simulink model "Logan"  (R2024b)
settings: Solver=ode4  StartTime=0  StopTime=inf  FixedStep=0.01  RelTol=1e-3
values from neighbouring files (symbols this model uses):
  AltPoint = 100000    [Logan_init.m]
  area_secao = 79.402*1.5    (= 119.103)    [Logan_init.m]
  b = 9    [Logan_init.m]
  c = 15.252    [Logan_init.m]
  cp = 1003    [Logan_init.m]
  E = 110e9    (= 110000000000)    [Logan_init.m]
  eta_comb = 0.95    [Logan_init.m]
  Fuel_Freeze = 0    [Logan_init.m]
  g = 9.80665    [Logan_init.m]
  gamma = 1.4    [Logan_init.m]
  GammaRef_deg = 0    [Logan_init.m]
  h1 = 0.5746    [Logan_init.m]
  h2 = 0.7752    [Logan_init.m]
  h3 = 0.1502    [Logan_init.m]
  hc = h1 + h2 + h3    (= 1.5)    [Logan_init.m]
  he = 2.6    [Logan_init.m]
  Inertia = [Ixx 0 -Ixz; 0 Iyy 0; -Ixz 0 Izz]    [Logan_init.m]
  L = 22.5    [Logan_init.m]
  L_inlet = 5.5    [Logan_init.m]
  La = 5    [Logan_init.m]
  LHV = 120 * 10^6    (= 120000000)    [Logan_init.m]
  Ln0 = 4.8    [Logan_init.m]
  MachPoint = 10    [Logan_init.m]
  Manual_Control = 0    [Logan_init.m]
  MW_air = 28.85    [Logan_init.m]
  MW_H2 = 2.00    (= 2)    [Logan_init.m]
  PA_EngineMode = 0    [Logan_init.m]
  PA_LatMode = 2    [Logan_init.m]
  PA_LongMode = 2    [Logan_init.m]
  PA_TECSEngineInput = 0    [Logan_init.m]
  PhiPoint = 0    [Logan_init.m]
  R = 287    [Logan_init.m]
  RefMass_kg = 31000    [Logan_init.m]
  S = 91.5    [Logan_init.m]
  tau1 = 3.1    [Logan_init.m]
  tau2 = 18.23    [Logan_init.m]
  TECS_ON = 0    [Logan_init.m]
  theta1 = 4    [Logan_init.m]
  theta2 = 6    [Logan_init.m]
  theta_n = 4    [Logan_init.m]
  ThetaPoint = 0    [Logan_init.m]
  Trimming = 0    [Logan_init.m]    (also in Logan_trim.m)
  w = 3.000    (= 3)    [Logan_init.m]
  Waypoint_idx = 1    [Logan_init.m]
  Waypoints = [ ... (first row only)    [Logan_init.m]
  x_a = 3.7    [Logan_init.m]
  x_inlet = 6    [Logan_init.m]
  x_n0 = 3    [Logan_init.m]
  xf_m = 0    [Logan_init.m]
  y_cg = 0    [Logan_init.m]
  z_a = 0.4    [Logan_init.m]
  z_cg = -0.996    [Logan_init.m]
  z_inlet = 0.7    [Logan_init.m]
  zf_m = 0    [Logan_init.m]
undefined symbols (not defined in the file or in its folder): Earth, Receive, Send, WGS84
libraries: simulink x4, spsFirstOrderFilterLib x4, aerolibactuator x3, aerolibfltsims x2, aerolibatmos2 x1, aerolibtransform2 x1, aerolibanimutils x1, dspswit3 x1, spsEdgeDetectorLib x1
(part 1 of 5)
settings Model: PacingRate=1000  Creator=bruno  LastModifiedBy=Ermer
settings SolverCC: NumberNewtonIterations=10  AlgebraicLoopSolver=TrustRegion
settings DataIOCC: ExternalInput=getinputstruct(opreport)  InitialState=getstatestruct(opreport)  LoadExternalInput=on  LoadInitialState=on  SaveFormat=StructureWithTime  ReturnWorkspaceOutputs=off
settings OptimizationCC: BlockReduction=off  DefaultParameterBehavior=Inlined  OptimizeBlockIOStorage=off  BufferReuse=off  EnhancedBackFolding=on  PassReuseOutputArgsAs=Individual arguments  ZeroExternalMemoryAtStartup=off  ZeroInternalMemoryAtStartup=off  OptimizeBlockOrder=speed  DifferentSizesBufferReuse=on  EfficientTunableParamExpr=on
settings DebuggingCC: AlgebraicLoopMsg=none  ParameterTunabilityLossMsg=error  SFUnexpectedBacktrackingDiag=warning  SFNoUnconditionalDefaultTransitionDiag=warning  ArithmeticOperatorsInVariantConditions=warning
settings ModelReferenceCC: EnableRefExpFcnMdlSchedulingChecks=on
settings SFSimCC: SimUseLocalCustomCode=off  MATLABDynamicMemAlloc=off  CustomCodeUndefinedFunction=UseInterfaceOnly
settings RTWCC: Description=Embedded Coder  SystemTargetFile=ert.tlc  TemplateMakefile=ert_default_tmf  RTWUseLocalCustomCode=off  GPUComputeCapability=3.5
settings CodeAppCC: ForceParamTrailComments=on  IgnoreCustomStorageClasses=off  OperatorAnnotations=on  SimulinkDataObjDesc=on  SFDataObjDesc=on  InsertBlockDesc=on
settings ERTTargetCC: GenerateSampleERTMain=on  SupportContinuousTime=on  ERTCustomFileTemplate=example_file_process.tlc  DynamicArrayContainerType=coder::array
settings ConfigComp: CovMetricSettings=dw  CovSaveCumulativeToWorkspaceVar=on  CovSaveSingleToWorkspaceVar=on  CovExternalEMLEnable=off
settings ExplorerConfigSet: SimMechanicsOpenEditorOnUpdate=off

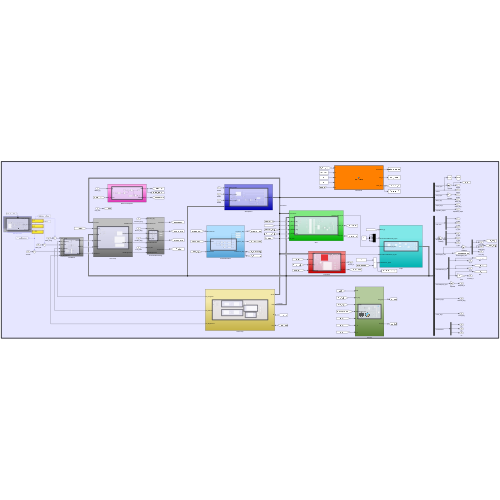
[thumbnail: Simulink's stored preview of the top-level diagram]
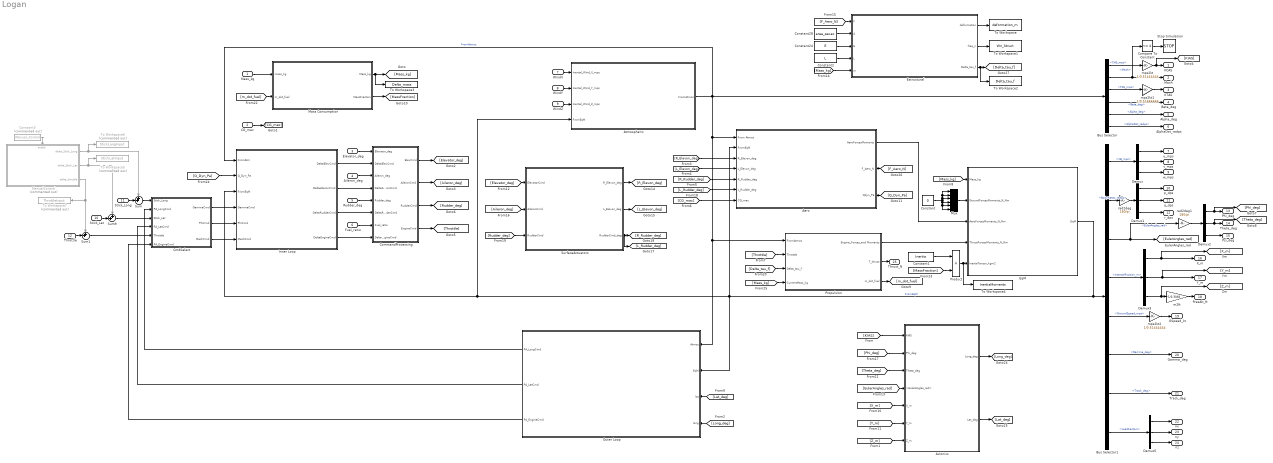
== system Logan ==
  Mass_kg : Inport  OutDataTypeStr=double
  CG_mac : Inport  Port=2  OutDataTypeStr=double
  Elevator_deg : Inport  Port=3  OutDataTypeStr=double
  Aileron_deg : Inport  Port=4  OutDataTypeStr=double
  Rudder_deg : Inport  Port=5  OutDataTypeStr=double
  Fuel_ratio : Inport  Port=6  OutDataTypeStr=double
  WindX : Inport  Port=7  OutDataTypeStr=double
  WindY : Inport  Port=8  OutDataTypeStr=double
  WindZ : Inport  Port=9  OutDataTypeStr=double
  Stick_Lat : Inport  Port=10
  Stick_Long : Inport  Port=11
  Throttle : Inport  Port=12  OutDataTypeStr=double
  Aero : Subsystem
  Atmospheric : Subsystem
  Avionics : Subsystem
  Bus Selector : BusSelector  OutputSignals=CAS_mps,Mach,TAS_mps,Beta_deg,Alpha_deg,AlphaDot_radps
  Bus Selector1 : BusSelector  OutputSignals=VB_mps,BodyRates_radps,EulerAngles_rad,IntertialPosition_m,GroundSpeed_mps,Gamma_deg,Track_deg,LoadFactors
  CmdSelect : Subsystem
  CommandProcessing : Subsystem
  Compare To Constant : simulink/Logic and Bit Operations/Compare To Constant  relop=<=  const=4  OutDataTypeStr=boolean
  Constant : Constant  Value=0  OutDataTypeStr=double
  Constant1 : Constant  Value=Inertia  OutDataTypeStr=double
  Constant2 : Constant  Value=L
  Constant24 : Constant  Value=E
  Constant28 : Constant  Value=area_secao
  Constant3 : Constant  Commented=on  Value=Manual_Control
  Demux{,1..3,5} (5 alike) : Demux  Outputs=3
  EqM : Subsystem
  Estructural : MATLAB Function  TreatAsAtomicUnit=on
  Inner Loop : Subsystem
  ManualControl : Subsystem  Commented=on
  Mass Consumption : Subsystem
  Mux : Mux  Inputs=6
  Outer Loop : Subsystem
  Product : Product
  Propulsion : Subsystem
  Stop Simulation : Stop
  Sum : Sum  Inputs=++|
  Sum1 : Sum  Inputs=++|
  Sum9 : Sum  Inputs=++|
  SurfaceActuators : Subsystem
  To Workspace : ToWorkspace  VariableName=deformation_m  SampleTime=-1
      settings: Save2DSignal=2-D array (concatenate along first dimension)
  To Workspace1 : ToWorkspace  VariableName=Wn_Struct  SampleTime=-1
      settings: Save2DSignal=2-D array (concatenate along first dimension)
  To Workspace2 : ToWorkspace  VariableName=Delta_tau_f  SampleTime=-1
  To Workspace3 : ToWorkspace  VariableName=Delta_mass  SampleTime=-1
      settings: Save2DSignal=2-D array (concatenate along first dimension)
  To Workspace4 : ToWorkspace  VariableName=InertiaMoments  SampleTime=-1
  To Workspace5 : ToWorkspace  Commented=on  VariableName=StickLatInput  SampleTime=-1
      settings: Save2DSignal=2-D array (concatenate along first dimension)
  To Workspace6 : ToWorkspace  Commented=on  VariableName=StickLongInput  SampleTime=-1
      settings: Save2DSignal=2-D array (concatenate along first dimension)
  To Workspace7 : ToWorkspace  Commented=on  VariableName=ThrottleInput  SampleTime=-1
      settings: Save2DSignal=2-D array (concatenate along first dimension)
  m2ft : Gain  Gain=-1/0.3048
  mps2kt : Gain  Gain=1/0.51444444
  mps2kt1 : Gain  Gain=1/0.51444444
  mps2kt2 : Gain  Gain=1/0.51444444
  rad2deg : Gain  Gain=180/pi
  rad2deg1 : Gain  Gain=180/pi
  KCAS : Outport
  Mach : Outport  Port=2
  KTAS : Outport  Port=3
  Beta_deg : Outport  Port=4
  Alpha_deg : Outport  Port=5
  AlphaDot_radps : Outport  Port=6
  u_mps : Outport  Port=7
  v_mps : Outport  Port=8
  w_mps : Outport  Port=9
  p_dps : Outport  Port=10
  q_dps : Outport  Port=11
  r_dps : Outport  Port=12
  Phi_deg : Outport  Port=13
  Theta_deg : Outport  Port=14
  Psi_deg : Outport  Port=15
  X_m : Outport  Port=16
  Y_m : Outport  Port=17
  PresAlt_ft : Outport  Port=18
  GSpeed_kt : Outport  Port=19
  Gamma_deg : Outport  Port=20
  Track_deg : Outport  Port=21
  nx : Outport  Port=22
  ny : Outport  Port=23
  nz : Outport  Port=24
  Thrust_N : Outport  Port=25
  wires:
  Atmospheric/1(FromAtmos) -> Outer Loop/1(Atmos), Propulsion/1(FromAtmos), Aero/1(From Atmos), Inner Loop/1(FromAtm), Bus Selector/1  "FromAtmos"
  Aero/1(AeroForcesMoments) -> EqM/3(AeroForcesMoments_N_Nm)
  Propulsion/1(Engine_Forces_and Moments) -> EqM/4(ThrustForcesMoments_N_Nm)
  EqM/1(EqM) -> Outer Loop/2(EqM), Inner Loop/3(FromEqM), Atmospheric/4(FromEqM), Aero/2(FromEqM), Bus Selector1/1  "FromEqM"
  Constant/1 -> Mux/4, Mux/5, Mux/6, Mux/2, Mux/1, Mux/3
  Mux/1 -> EqM/2(GroundForcesMoments_N_Nm)
  CG_mac/1 -> [CG_mac]
  WindX/1 -> Atmospheric/1(Inertial_Wind_X_mps)
  WindY/1 -> Atmospheric/2(Inertial_Wind_Y_mps)
  WindZ/1 -> Atmospheric/3(Inertial_Wind_Z_mps)
  [R_Elevon_deg] -> Aero/3(R_Elevon_deg)
  [L_Elevon_deg] -> Aero/4(L_Elevon_deg)
  [R_Rudder_deg] -> Aero/5(R_Rudder_deg)
  [CG_mac] -> Aero/7(CG_mac)
  [Mass_kg] -> EqM/1(Mass_kg)
  Propulsion/2(T_thrust) -> Thrust_N/1
  Bus Selector/1 -> mps2kt/1  "<CAS_mps>"
  Bus Selector/2 -> Compare To Constant/1, Mach/1  "<Mach>"
  Bus Selector/3 -> mps2kt1/1  "<TAS_mps>"
  mps2kt1/1 -> KTAS/1
  Bus Selector/4 -> Beta_deg/1  "<Beta_deg>"
  Bus Selector/5 -> Alpha_deg/1  "<Alpha_deg>"
  Bus Selector/6 -> AlphaDot_radps/1  "<AlphaDot_radps>"
  Bus Selector1/1 -> Demux/1  "<VB_mps>"
  Demux/1 -> u_mps/1
  Demux/2 -> v_mps/1
  Demux/3 -> w_mps/1
  Bus Selector1/2 -> rad2deg/1  "<BodyRates_radps>"
  Demux1/1 -> p_dps/1
  Demux1/3 -> r_dps/1
  Bus Selector1/3 -> rad2deg1/1, [EulerAngles_rad]  "<EulerAngles_rad>"
  Demux2/2 -> Theta_deg/1, [Theta_deg]
  Demux2/3 -> Psi_deg/1
  rad2deg/1 -> Demux1/1
  rad2deg1/1 -> Demux2/1
  Bus Selector1/4 -> Demux3/1  "<IntertialPosition_m>"
  Demux3/1 -> X_m/1, [X_m]
  Demux3/2 -> Y_m/1, [Y_m]
  Demux3/3 -> [Z_m], m2ft/1
  m2ft/1 -> PresAlt_ft/1
  Bus Selector1/5 -> mps2kt2/1  "<GroundSpeed_mps>"
  mps2kt2/1 -> GSpeed_kt/1
  Bus Selector1/6 -> Gamma_deg/1  "<Gamma_deg>"
  Bus Selector1/7 -> Track_deg/1  "<Track_deg>"
  Bus Selector1/8 -> Demux5/1  "<LoadFactors>"
  Demux5/1 -> nx/1
  Demux5/2 -> ny/1
  Demux5/3 -> nz/1
  [Throttle] -> Propulsion/2(Throttle)
  mps2kt/1 -> KCAS/1, [KIAS]
  Demux1/2 -> q_dps/1
  [L_Rudder_deg] -> Aero/6(L_Rudder_deg)
  Estructural/1(deformation) -> To Workspace/1
  Estructural/2(freq_n) -> To Workspace1/1
  Avionics/1(Long_deg) -> [Long_deg]
  Avionics/2(Lat_deg) -> [Lat_deg]
  [Mass_kg] -> Estructural/5(m)
  Constant2/1 -> Estructural/4(L)
  Constant24/1 -> Estructural/3(E)
  Constant28/1 -> Estructural/2(A)
  Aero/2(F_Aero_N) -> [F_Aero_N]
  [F_Aero_N] -> Estructural/1(F)
  Estructural/3(Delta_tau_f) -> To Workspace2/1, [Delta_tau_f]
  [Delta_tau_f] -> Propulsion/3(Delta_tau_f)
  SurfaceActuators/1(R_Elevon_deg) -> [R_Elevon_deg]
  SurfaceActuators/2(L_Elevon_deg) -> [L_Elevon_deg]
  [Aileron_deg] -> SurfaceActuators/2(AileronCmd)
  [Elevator_deg] -> SurfaceActuators/1(ElevatorCmd)
  [Rudder_deg] -> SurfaceActuators/3(RudderCmd)
  SurfaceActuators/3(RudderCmd_deg) -> [R_Rudder_deg], [L_Rudder_deg]
  Elevator_deg/1 -> CommandProcessing/1(Elevator_deg)
  Inner Loop/1(DeltaElevCmd) -> CommandProcessing/2(DeltaElevCmd)
  CmdSelect/1(GammaCmd) -> Inner Loop/4(GammaCmd)
  Constant3/1 -> ManualControl/Enable
  Stick_Long/1 -> Sum/2
  Sum/1 -> CmdSelect/1(Stick_Long)
  ManualControl/1(delta_Stick_Long) -> To Workspace6/1, Sum/1
  Inner Loop/2(DeltaAileronCmd) -> CommandProcessing/4(DeltaAileronCmd)
  Inner Loop/3(DeltaRudderCmd) -> CommandProcessing/6(DeltaRudderCmd)
  CommandProcessing/3(RudderCmd) -> [Rudder_deg]
  Rudder_deg/1 -> CommandProcessing/5(Rudder_deg)
  CommandProcessing/2(AileronCmd) -> [Aileron_deg]
  Aileron_deg/1 -> CommandProcessing/3(Aileron_deg)
  Sum9/1 -> CmdSelect/3(Stick_Lat)
  Stick_Lat/1 -> Sum9/2
  ManualControl/2(delta_Stick_Lat) -> To Workspace5/1, Sum9/1
  CmdSelect/2(PhiCmd) -> Inner Loop/5(PhiCmd)
  CmdSelect/3(MachCmd) -> Inner Loop/6(MachCmd)
  ManualControl/3(delta_throttle) -> Sum1/1, To Workspace7/1
  Sum1/1 -> CmdSelect/5(Throttle)
  Outer Loop/1(PA_LongCmd) -> CmdSelect/2(PA_LongCmd)
  Outer Loop/2(PA_LatCmd) -> CmdSelect/4(PA_LatCmd)
  [Lat_deg] -> Outer Loop/3(lat)
  [Long_deg] -> Outer Loop/4(long)
  [Z_m] -> Avionics/7(Z_m)
  [KIAS] -> Avionics/1(KIAS)
  [X_m] -> Avionics/5(X_m)
  [Y_m] -> Avionics/6(Y_m)
  [EulerAngles_rad] -> Avionics/4(<EulerAngles_rad>)
  [Phi_deg] -> Avionics/2(Phi_deg)
  [Theta_deg] -> Avionics/3(Theta_deg)
  Demux2/1 -> Phi_deg/1, [Phi_deg]
  Outer Loop/3(PA_EngineCmd) -> CmdSelect/6(PA_EngineCmd)
  Throttle/1 -> Sum1/2
  CommandProcessing/4(EngineCmd) -> [Throttle]
  Inner Loop/4(DeltaEngineCmd) -> CommandProcessing/8(DeltaEngineCmd)
  Fuel_ratio/1 -> CommandProcessing/7(Fuel_ratio)
  CommandProcessing/1(ElevCmd) -> [Elevator_deg]
  Propulsion/3(m_dot_fuel) -> [m_dot_fuel]
  Mass_kg/1 -> Mass Consumption/1(mass_kg)
  Mass Consumption/1(Mass_kg) -> To Workspace3/1, [Mass_kg]
  [m_dot_fuel] -> Mass Consumption/2(m_dot_fuel)
  Mass Consumption/2(MassFraction) -> [MassFraction]
  Product/1 -> To Workspace4/1, EqM/5(InertiaTensor_kgm2)
  Constant1/1 -> Product/1
  [MassFraction] -> Product/2
  [Mass_kg] -> Propulsion/4(CurrentMass_kg)
  Compare To Constant/1 -> Stop Simulation/1
  Aero/3(Qdyn_Pa) -> [Q_Dyn_Pa]
  [Q_Dyn_Pa] -> Inner Loop/2(Q_Dyn_Pa)

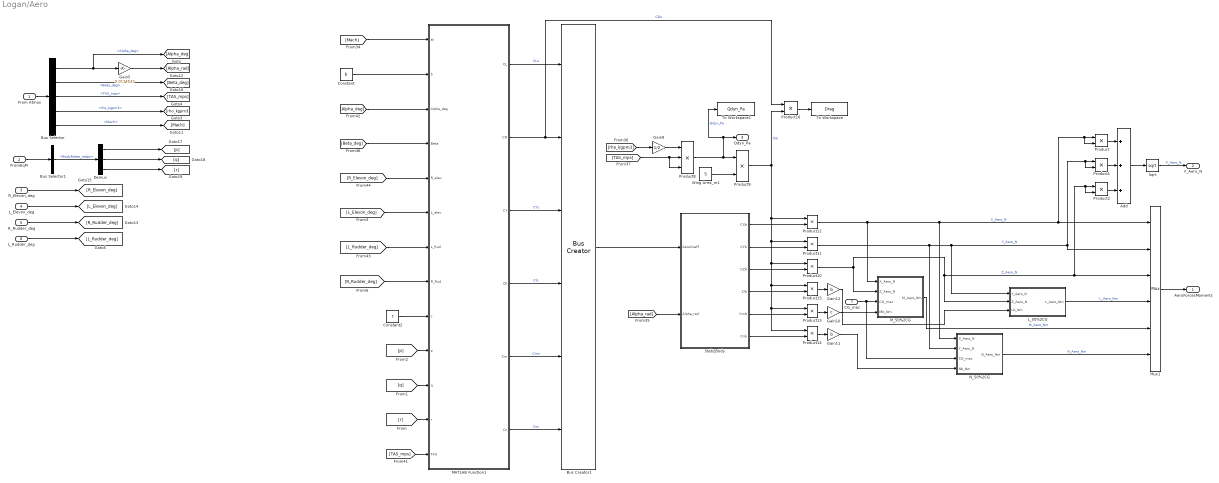
== system Logan/Aero ==
  From Atmos : Inport
  FromEqM : Inport  Port=2
  R_Elevon_deg : Inport  Port=3
  L_Elevon_deg : Inport  Port=4
  R_Rudder_deg : Inport  Port=5
  L_Rudder_deg : Inport  Port=6
  CG_mac : Inport  Port=7
  Add : Sum  Inputs=+++
  Bus Creator1 : BusCreator  Inputs=6
  Bus Selector : BusSelector  OutputSignals=Alpha_deg,Beta_deg,TAS_mps,rho_kgpm3,Mach
  Bus Selector1 : BusSelector  OutputSignals=BodyRates_radps
  Constant : Constant  Value=b
  Constant2 : Constant  Value=c
  Demux : Demux  Outputs=3
  Gain10 : Gain  Gain=c
  Gain11 : Gain  Gain=b
  Gain12 : Gain  Gain=b
  Gain5 : Gain  Gain=0.0174533
  Gain9 : Gain  Gain=1/2
  L_50%2CG : Subsystem
  MATLAB Function1 : MATLAB Function  TreatAsAtomicUnit=on
  M_50%2CG : Subsystem
  Mux1 : Mux  Inputs=6
  N_50%2CG : Subsystem
  Product{,1..2,9..16} (11 alike) : Product
  Product8 : Product  Inputs=3
  Sqrt : Sqrt
  Stab2Body : Subsystem
  To Workspace : ToWorkspace  VariableName=Drag  SampleTime=-1
      settings: Save2DSignal=2-D array (concatenate along first dimension)
  To Workspace1 : ToWorkspace  VariableName=Qdyn_Pa  SampleTime=-1
      settings: Save2DSignal=2-D array (concatenate along first dimension)
  Wing Area_m1 : Constant  Value=S
  AeroForcesMoments : Outport
  F_Aero_N : Outport  Port=2
  Qdyn_Pa : Outport  Port=3
  wires:
  Bus Selector/4 -> [rho_kgpm3]  "<rho_kgpm3>"
  Bus Selector/3 -> [TAS_mps]  "<TAS_mps>"
  R_Rudder_deg/1 -> [R_Rudder_deg]
  Bus Selector/2 -> [Beta_deg]  "<Beta_deg>"
  L_Elevon_deg/1 -> [L_Elevon_deg]
  From Atmos/1 -> Bus Selector/1
  Bus Selector/1 -> [Alpha_deg], Gain5/1  "<Alpha_deg>"
  FromEqM/1 -> Bus Selector1/1
  Bus Selector1/1 -> Demux/1  "<BodyRates_radps>"
  Bus Selector/5 -> [Mach]  "<Mach>"
  Gain5/1 -> [Alpha_rad]
  Product15/1 -> Gain12/1
  Wing Area_m1/1 -> Product9/2
  Product10/1 -> M_50%2CG/2(Z_Aero_N), L_50%2CG/2(Z_Aero_N), Product2/2, Product2/1, Mux1/3  "Z_Aero_N"
  Product9/1 -> Product16/2, Product10/1, Product13/1, Product14/1, Product15/1, Product11/1, Product12/1  "QS"
  CG_mac/1 -> M_50%2CG/3(CG_mac), N_50%2CG/3(CG_mac)
  Product11/1 -> N_50%2CG/2(Y_Aero_N), Product1/2, Product1/1, Mux1/2, L_50%2CG/1(Y_Aero_N)  "Y_Aero_N"
  L_50%2CG/1(L_Aero_Nm) -> Mux1/4  "L_Aero_Nm"
  Product8/1 -> To Workspace1/1, Qdyn_Pa/1, Product9/1  "Qdyn_Pa"
  [TAS_mps] -> Product8/2, Product8/3
  Gain9/1 -> Product8/1
  Gain11/1 -> N_50%2CG/4(Nb_Nm)
  Product14/1 -> Gain11/1
  M_50%2CG/1(M_Aero_Nm) -> Mux1/5  "M_Aero_Nm"
  [rho_kgpm3] -> Gain9/1
  Product12/1 -> M_50%2CG/1(X_Aero_N), N_50%2CG/1(X_Aero_N), Product/2, Product/1, Mux1/1  "X_Aero_N"
  Gain10/1 -> M_50%2CG/4(Mb_Nm)
  Product13/1 -> Gain10/1
  Gain12/1 -> L_50%2CG/3(Lb_Nm)
  N_50%2CG/1(N_Aero_Nm) -> Mux1/6  "N_Aero_Nm"
  [TAS_mps] -> MATLAB Function1/13(TAS)
  [Mach] -> MATLAB Function1/1(M)
  Constant/1 -> MATLAB Function1/2(b)
  Constant2/1 -> MATLAB Function1/9(c)
  MATLAB Function1/2(CD) -> Product16/1, Bus Creator1/2  "CDs"
  MATLAB Function1/3(CY) -> Bus Creator1/3  "CYs"
  MATLAB Function1/4(Cll) -> Bus Creator1/4  "Cls"
  MATLAB Function1/5(Cm) -> Bus Creator1/5  "Cms"
  MATLAB Function1/6(Cn) -> Bus Creator1/6  "Cns"
  MATLAB Function1/1(CL) -> Bus Creator1/1  "CLs"
  Mux1/1 -> AeroForcesMoments/1
  R_Elevon_deg/1 -> [R_Elevon_deg]
  Product16/1 -> To Workspace/1
  [Alpha_rad] -> Stab2Body/2(Alpha_rad)
  Demux/1 -> [p]
  Demux/2 -> [q]
  Demux/3 -> [r]
  L_Rudder_deg/1 -> [L_Rudder_deg]
  Stab2Body/6(Cnb) -> Product14/2
  Stab2Body/5(Cmb) -> Product13/2
  Stab2Body/4(Clb) -> Product15/2
  Stab2Body/3(CZb) -> Product10/2
  Stab2Body/2(CYb) -> Product11/2
  Stab2Body/1(CXb) -> Product12/2
  Bus Creator1/1 -> Stab2Body/1(AeroCoeff)
  [r] -> MATLAB Function1/12(r)
  [Beta_deg] -> MATLAB Function1/4(Beta)
  [q] -> MATLAB Function1/11(q)
  [p] -> MATLAB Function1/10(p)
  [Alpha_deg] -> MATLAB Function1/3(Alpha_deg)
  [R_Elevon_deg] -> MATLAB Function1/5(R_elev)
  [L_Elevon_deg] -> MATLAB Function1/6(L_elev)
  [L_Rudder_deg] -> MATLAB Function1/7(L_Rud)
  [R_Rudder_deg] -> MATLAB Function1/8(R_Rud)
  Add/1 -> Sqrt/1
  Product/1 -> Add/1
  Product1/1 -> Add/2
  Product2/1 -> Add/3
  Sqrt/1 -> F_Aero_N/1  "F_Aero_N"

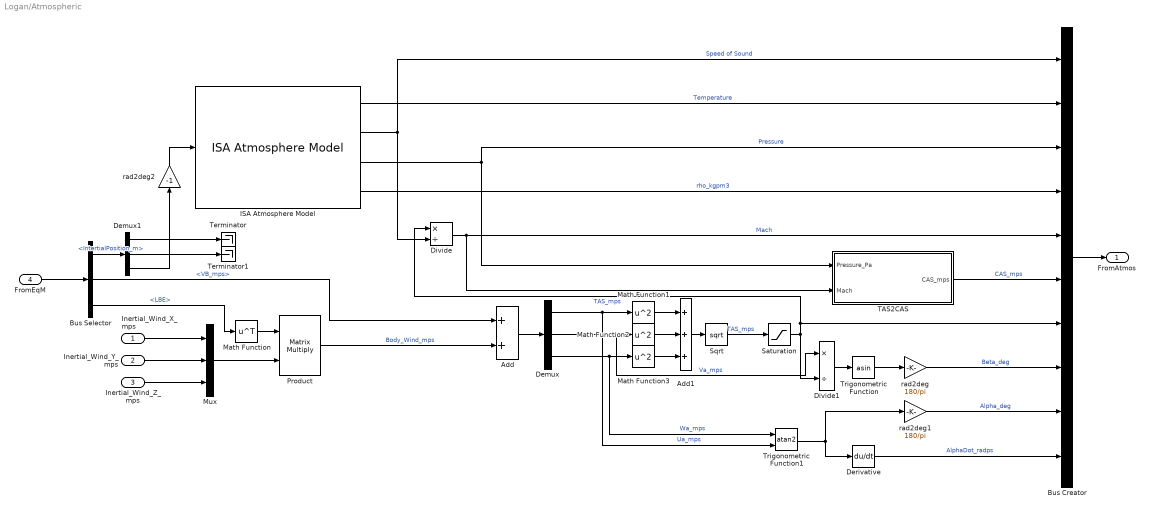
== system Logan/Atmospheric ==
  Inertial_Wind_X_mps : Inport
  Inertial_Wind_Y_mps : Inport  Port=2
  Inertial_Wind_Z_mps : Inport  Port=3
  FromEqM : Inport  Port=4
  Add : Sum
  Add1 : Sum  Inputs=+++
  Bus Creator : BusCreator  Inputs=10
  Bus Selector : BusSelector  OutputSignals=IntertialPosition_m,VB_mps,LBE
  Demux : Demux  Outputs=3
  Demux1 : Demux  Outputs=3
  Derivative : Derivative
  Divide : Product  Inputs=*/
  Divide1 : Product  Inputs=*/
  ISA Atmosphere Model : aerolibatmos2/ISA Atmosphere Model  useExtended=on  action=Warning  custom=off  viscosityOut=off  g=9.80665  gamma=1.4  R=287.0531  L=0.0065  h_trop=11000  h_strat=20000  rho0=1.225  P0=101325  T0=288.15  h0=0  S=110.4  Tref=273.15  muref=1.716e-5
  Math Function : Math  Operator=transpose  SignedPower=on
  Math Function1 : Math  Operator=square  SignedPower=on
  Math Function2 : Math  Operator=square  SignedPower=on
  Math Function3 : Math  Operator=square  SignedPower=on
  Mux : Mux  Inputs=3
  Product : Product  Multiplication=Matrix(*)
  Saturation : Saturate  UpperLimit=inf  LowerLimit=1
  Sqrt : Sqrt
  TAS2CAS : Subsystem
  Terminator : Terminator
  Terminator1 : Terminator
  Trigonometric Function : Trigonometry  Operator=asin
  Trigonometric Function1 : Trigonometry  Operator=atan2
  rad2deg : Gain  Gain=180/pi
  rad2deg1 : Gain  Gain=180/pi
  rad2deg2 : Gain  Gain=-1
  FromAtmos : Outport
  wires:
  rad2deg/1 -> Bus Creator/8  "Beta_deg"
  Math Function3/1 -> Add1/3
  Add1/1 -> Sqrt/1
  Math Function1/1 -> Add1/1
  Demux/2 -> Math Function2/1, Divide1/1  "Va_mps"
  Demux/3 -> Math Function3/1, Trigonometric Function1/1  "Wa_mps"
  Divide1/1 -> Trigonometric Function/1
  Trigonometric Function/1 -> rad2deg/1
  Math Function2/1 -> Add1/2
  Demux/1 -> Math Function1/1, Trigonometric Function1/2  "Ua_mps"
  Add/1 -> Demux/1
  Demux1/3 -> rad2deg2/1
  TAS2CAS/1(CAS_mps) -> Bus Creator/6  "CAS_mps"
  Product/1 -> Add/2  "Body_Wind_mps"
  Mux/1 -> Product/2
  Math Function/1 -> Product/1
  Inertial_Wind_Z_mps/1 -> Mux/3
  Sqrt/1 -> Saturation/1  "TAS_mps"
  FromEqM/1 -> Bus Selector/1
  Divide/1 -> TAS2CAS/2(Mach), Bus Creator/5  "Mach"
  Inertial_Wind_X_mps/1 -> Mux/1
  Inertial_Wind_Y_mps/1 -> Mux/2
  rad2deg1/1 -> Bus Creator/9  "Alpha_deg"
  Bus Creator/1 -> FromAtmos/1
  Trigonometric Function1/1 -> Derivative/1, rad2deg1/1
  Derivative/1 -> Bus Creator/10  "AlphaDot_radps"
  Bus Selector/3 -> Math Function/1  "<LBE>"
  Bus Selector/2 -> Add/1  "<VB_mps>"
  Bus Selector/1 -> Demux1/1  "<IntertialPosition_m>"
  Demux1/1 -> Terminator/1
  Demux1/2 -> Terminator1/1
  rad2deg2/1 -> ISA Atmosphere Model/1
  Saturation/1 -> Divide/1, Bus Creator/7, Divide1/2  "TAS_mps"
  ISA Atmosphere Model/1 -> Bus Creator/2  "Temperature"
  ISA Atmosphere Model/2 -> Bus Creator/1, Divide/2  "Speed of Sound"
  ISA Atmosphere Model/3 -> Bus Creator/3, TAS2CAS/1(Pressure_Pa)  "Pressure"
  ISA Atmosphere Model/4 -> Bus Creator/4  "rho_kgpm3"

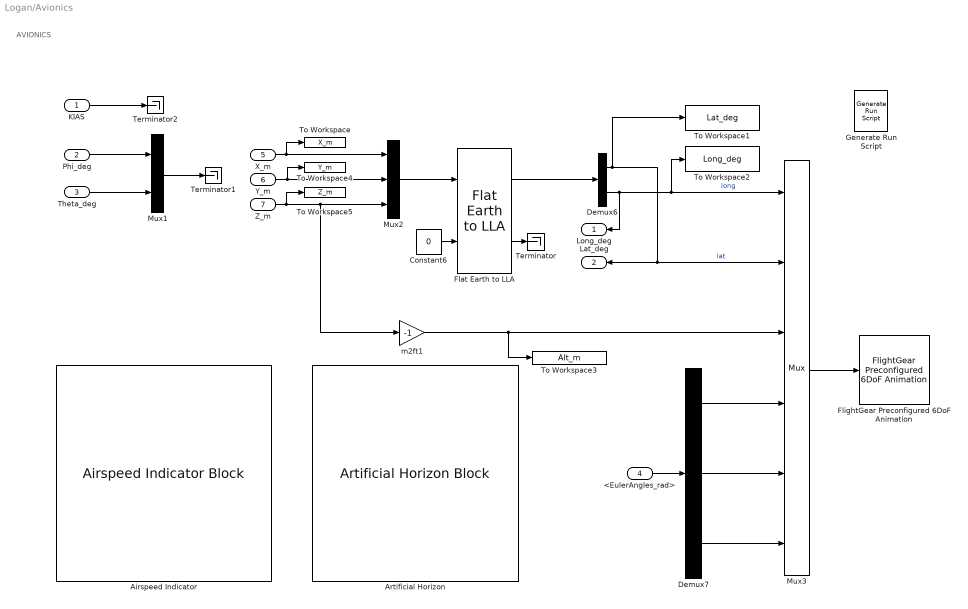
== system Logan/Avionics ==
  note: AVIONICS
  KIAS : Inport
  Phi_deg : Inport  Port=2
  Theta_deg : Inport  Port=3
  <EulerAngles_rad> : Inport  Port=4
  X_m : Inport  Port=5
  Y_m : Inport  Port=6
  Z_m : Inport  Port=7
  Airspeed Indicator : AirspeedIndicatorBlock  LabelPosition=Hide  ScaleMin=0  ScaleMax=7000
  Artificial Horizon : ArtificialHorizonBlock  LabelPosition=Hide
  Constant6 : Constant  Value=0
  Demux6 : Demux  Outputs=2
  Demux7 : Demux  Outputs=3
  Flat Earth to LLA : aerolibtransform2/Flat Earth to LLA  units=Metric (MKS)  ptype=Earth (WGS84)  F=1/298.257223563  R=6378137  refPosPort=off  LL0=[-23.5505 -46.6333]  psi=0
  FlightGear Preconfigured 6DoF Animation : aerolibfltsims/FlightGear Preconfigured 6DoF Animation  xFlightGearVersion=v2019.1  DestinationIpAddress=127.0.0.1  DestinationPort=5502  SampleTime=-1  packetVersion=24
  Generate Run Script : aerolibfltsims/Generate Run Script  Architecture=Win64  dataFlow=Send-Receive  GeometryModelName=GHV  AirportId=KSFO  RunwayId=10L  InitialAltitude=7224  InitialHeading=113  OffsetDistance=4.72  OffsetAzimuth=0  InstallScenery=on  DisableShaders=off  OriginAddress=127.0.0.1  DestinationPort=5502  OriginPort=5505  LocalAddress=127.0.0.1  OutputFileName=runfg.bat  FlightGearBaseDirectory=C:\FlightGear 2020.3
  Mux1 : Mux  Inputs=2
  Mux2 : Mux  Inputs=3
  Mux3 : Mux  Inputs=6
  Terminator : Terminator
  Terminator1 : Terminator
  Terminator2 : Terminator
  To Workspace : ToWorkspace  VariableName=X_m  SampleTime=-1
      settings: Save2DSignal=2-D array (concatenate along first dimension)
  To Workspace1 : ToWorkspace  VariableName=Lat_deg  SampleTime=-1
  To Workspace2 : ToWorkspace  VariableName=Long_deg  SampleTime=-1
  To Workspace3 : ToWorkspace  VariableName=Alt_m  SampleTime=-1
  To Workspace4 : ToWorkspace  VariableName=Y_m  SampleTime=-1
      settings: Save2DSignal=2-D array (concatenate along first dimension)
  To Workspace5 : ToWorkspace  VariableName=Z_m  SampleTime=-1
      settings: Save2DSignal=2-D array (concatenate along first dimension)
  m2ft1 : Gain  Gain=-1
  Long_deg : Outport
  Lat_deg : Outport  Port=2
  wires:
  Z_m/1 -> m2ft1/1, Mux2/3, To Workspace5/1
  X_m/1 -> To Workspace/1, Mux2/1
  Y_m/1 -> To Workspace4/1, Mux2/2
  Demux6/2 -> Mux3/1, To Workspace2/1, Long_deg/1  "long"
  Demux7/2 -> Mux3/5
  Demux7/1 -> Mux3/4
  Flat Earth to LLA/1 -> Demux6/1
  Constant6/1 -> Flat Earth to LLA/2
  Demux7/3 -> Mux3/6
  Mux2/1 -> Flat Earth to LLA/1
  m2ft1/1 -> Mux3/3, To Workspace3/1
  Demux6/1 -> Lat_deg/1, Mux3/2, To Workspace1/1  "lat"
  <EulerAngles_rad>/1 -> Demux7/1
  Flat Earth to LLA/2 -> Terminator/1
  Mux1/1 -> Terminator1/1
  Phi_deg/1 -> Mux1/1
  Theta_deg/1 -> Mux1/2
  KIAS/1 -> Terminator2/1
  Mux3/1 -> FlightGear Preconfigured 6DoF Animation/1

== system Logan/CmdSelect ==
  Stick_Long : Inport
  PA_LongCmd : Inport  Port=2
  Stick_Lat : Inport  Port=3
  PA_LatCmd : Inport  Port=4
  Throttle : Inport  Port=5  OutDataTypeStr=double
  PA_EngineCmd : Inport  Port=6
  Constant : Constant  Value=PA_EngineMode
  Sum : Sum  Inputs=|++
  Sum1 : Sum  Inputs=|++
  Switch : Switch  Criteria=u2 > Threshold  SaturateOnIntegerOverflow=off  InputSameDT=off
  GammaCmd : Outport
  PhiCmd : Outport  Port=2
  MachCmd : Outport  Port=3
  wires:
  Stick_Long/1 -> Sum/1
  Sum/1 -> GammaCmd/1
  PA_LongCmd/1 -> Sum/2
  Stick_Lat/1 -> Sum1/1
  Sum1/1 -> PhiCmd/1
  PA_LatCmd/1 -> Sum1/2
  Constant/1 -> Switch/2
  Switch/1 -> MachCmd/1
  PA_EngineCmd/1 -> Switch/1
  Throttle/1 -> Switch/3

== system Logan/CommandProcessing ==
  Elevator_deg : Inport
  DeltaElevCmd : Inport  Port=2
  Aileron_deg : Inport  Port=3
  DeltaAileronCmd : Inport  Port=4
  Rudder_deg : Inport  Port=5  OutDataTypeStr=double
  DeltaRudderCmd : Inport  Port=6
  Fuel_ratio : Inport  Port=7  OutDataTypeStr=double
  DeltaEngineCmd : Inport  Port=8
  Saturation1 : Saturate  UpperLimit=30  LowerLimit=-25
  Saturation2 : Saturate  UpperLimit=25  LowerLimit=-25
  Sum{1..3,5} (4 alike) : Sum  Inputs=|++
  To Workspace1 : ToWorkspace  VariableName=Elevator_Demand  SampleTime=-1
      settings: Save2DSignal=2-D array (concatenate along first dimension)
  To Workspace2 : ToWorkspace  VariableName=Rudder_Demand  SampleTime=-1
      settings: Save2DSignal=2-D array (concatenate along first dimension)
  To Workspace33 : ToWorkspace  VariableName=Aileron_Demand  SampleTime=-1
      settings: Save2DSignal=2-D array (concatenate along first dimension)
  ElevCmd : Outport
  AileronCmd : Outport  Port=2
  RudderCmd : Outport  Port=3
  EngineCmd : Outport  Port=4
  wires:
  Sum5/1 -> To Workspace1/1, Saturation1/1
  Saturation1/1 -> ElevCmd/1
  Elevator_deg/1 -> Sum5/1
  DeltaElevCmd/1 -> Sum5/2
  Saturation2/1 -> AileronCmd/1
  Sum1/1 -> To Workspace33/1, Saturation2/1
  Aileron_deg/1 -> Sum1/1
  DeltaAileronCmd/1 -> Sum1/2
  Rudder_deg/1 -> Sum2/1
  Sum2/1 -> RudderCmd/1, To Workspace2/1
  DeltaRudderCmd/1 -> Sum2/2
  Fuel_ratio/1 -> Sum3/1
  Sum3/1 -> EngineCmd/1
  DeltaEngineCmd/1 -> Sum3/2

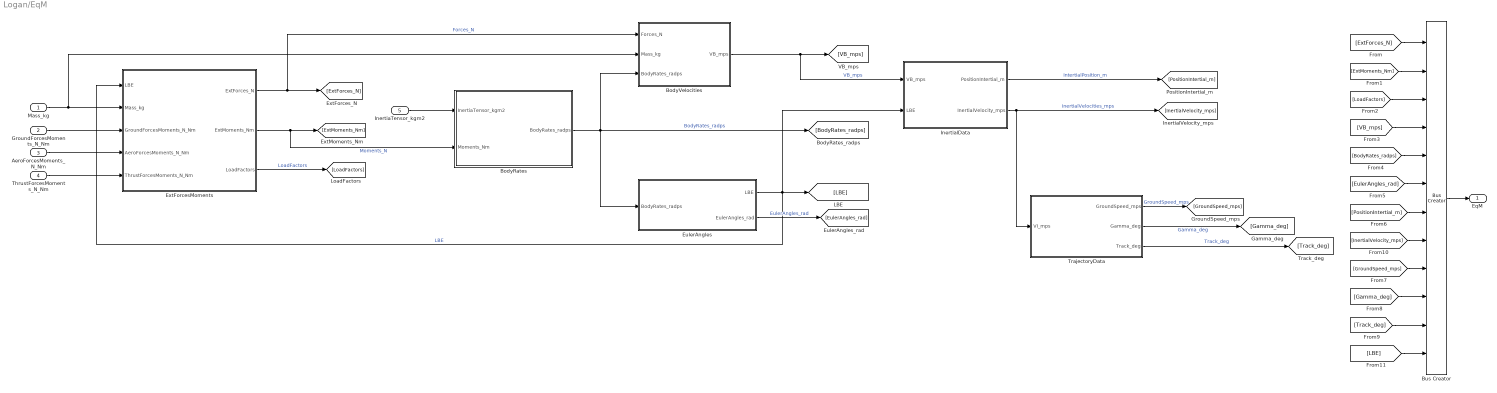
== system Logan/EqM ==
  Mass_kg : Inport
  GroundForcesMoments_N_Nm : Inport  Port=2
  AeroForcesMoments_N_Nm : Inport  Port=3
  ThrustForcesMoments_N_Nm : Inport  Port=4
  InertiaTensor_kgm2 : Inport  Port=5
  BodyRates : Subsystem
  BodyVelocities : Subsystem
  Bus Creator : BusCreator  Inputs=12
  EulerAngles : Subsystem
  ExtForcesMoments : Subsystem
  InertialData : Subsystem
  TrajectoryData : Subsystem
  EqM : Outport
  wires:
  [PositionIntertial_m] -> Bus Creator/7
  [EulerAngles_rad] -> Bus Creator/6
  [BodyRates_radps] -> Bus Creator/5
  [VB_mps] -> Bus Creator/4
  [ExtForces_N] -> Bus Creator/1
  Bus Creator/1 -> EqM/1
  [Track_deg] -> Bus Creator/11
  [ExtMoments_Nm] -> Bus Creator/2
  [Gamma_deg] -> Bus Creator/10
  [GroundSpeed_mps] -> Bus Creator/9
  TrajectoryData/1(GroundSpeed_mps) -> [GroundSpeed_mps]  "GroundSpeed_mps"
  EulerAngles/2(EulerAngles_rad) -> [EulerAngles_rad]  "EulerAngles_rad"
  TrajectoryData/3(Track_deg) -> [Track_deg]  "Track_deg"
  TrajectoryData/2(Gamma_deg) -> [Gamma_deg]  "Gamma_deg"
  AeroForcesMoments_N_Nm/1 -> ExtForcesMoments/4(AeroForcesMoments_N_Nm)
  ExtForcesMoments/3(LoadFactors) -> [LoadFactors]  "LoadFactors"
  Mass_kg/1 -> ExtForcesMoments/2(Mass_kg), BodyVelocities/2(Mass_kg)
  ExtForcesMoments/1(ExtForces_N) -> BodyVelocities/1(Forces_N), [ExtForces_N]  "Forces_N"
  BodyVelocities/1(VB_mps) -> InertialData/1(VB_mps), [VB_mps]  "VB_mps"
  EulerAngles/1(LBE) -> [LBE], ExtForcesMoments/1(LBE), InertialData/2(LBE)  "LBE"
  GroundForcesMoments_N_Nm/1 -> ExtForcesMoments/3(GroundForcesMoments_N_Nm)
  ThrustForcesMoments_N_Nm/1 -> ExtForcesMoments/5(ThrustForcesMoments_N_Nm)
  BodyRates/1(BodyRates_radps) -> BodyVelocities/3(BodyRates_radps), EulerAngles/1(BodyRates_radps), [BodyRates_radps]  "BodyRates_radps"
  InertiaTensor_kgm2/1 -> BodyRates/1(InertiaTensor_kgm2)
  ExtForcesMoments/2(ExtMoments_Nm) -> BodyRates/2(Moments_Nm), [ExtMoments_Nm]  "Moments_N"
  [InertialVelocity_mps] -> Bus Creator/8
  [LoadFactors] -> Bus Creator/3
  InertialData/2(InertialVelocity_mps) -> TrajectoryData/1(VI_mps), [InertialVelocity_mps]  "InertialVelocities_mps"
  InertialData/1(PositionIntertial_m) -> [PositionIntertial_m]  "IntertialPosition_m"
  [LBE] -> Bus Creator/12

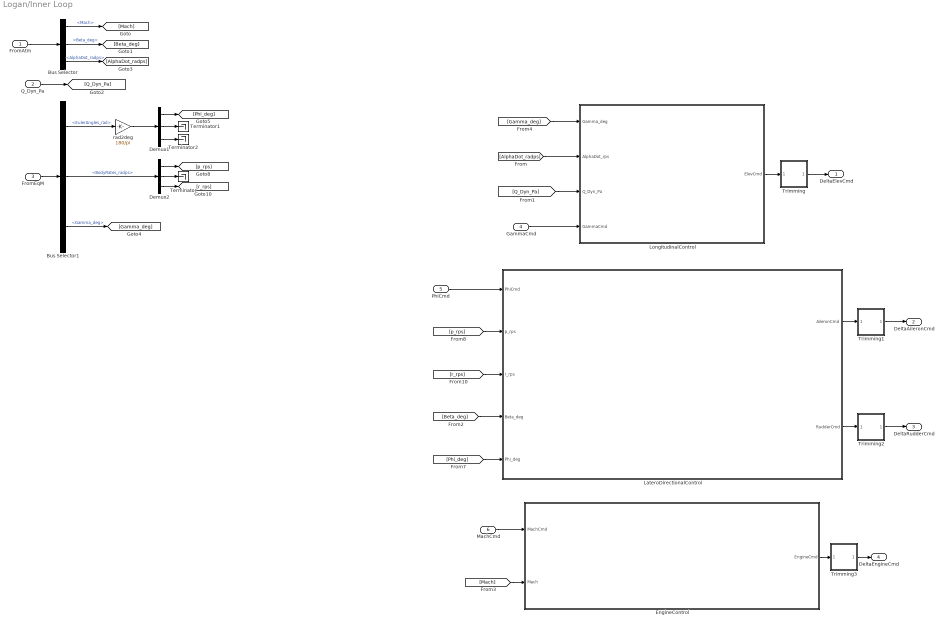
== system Logan/Inner Loop ==
  FromAtm : Inport
  Q_Dyn_Pa : Inport  Port=2
  FromEqM : Inport  Port=3
  GammaCmd : Inport  Port=4  OutDataTypeStr=double
  PhiCmd : Inport  Port=5  OutDataTypeStr=double
  MachCmd : Inport  Port=6  OutDataTypeStr=double
  Bus Selector : BusSelector  OutputSignals=Mach,Beta_deg,AlphaDot_radps
  Bus Selector1 : BusSelector  OutputSignals=EulerAngles_rad,BodyRates_radps,Gamma_deg
  Demux1 : Demux  Outputs=3
  Demux2 : Demux  Outputs=3
  EngineControl : Subsystem
  LateroDirectionalControl : Subsystem
  LongitudinalControl : Subsystem
  Terminator : Terminator
  Terminator1 : Terminator
  Terminator2 : Terminator
  Trimming : Subsystem
  Trimming1 : Subsystem
  Trimming2 : Subsystem
  Trimming3 : Subsystem
  rad2deg : Gain  Gain=180/pi
  DeltaElevCmd : Outport
  DeltaAileronCmd : Outport  Port=2
  DeltaRudderCmd : Outport  Port=3
  DeltaEngineCmd : Outport  Port=4
  wires:
  FromAtm/1 -> Bus Selector/1
  Bus Selector/1 -> [Mach]  "<Mach>"
  Bus Selector/2 -> [Beta_deg]  "<Beta_deg>"
  Bus Selector/3 -> [AlphaDot_radps]  "<AlphaDot_radps>"
  FromEqM/1 -> Bus Selector1/1
  rad2deg/1 -> Demux1/1
  Bus Selector1/1 -> rad2deg/1  "<EulerAngles_rad>"
  Bus Selector1/2 -> Demux2/1  "<BodyRates_radps>"
  Bus Selector1/3 -> [Gamma_deg]  "<Gamma_deg>"
  Demux1/1 -> [Phi_deg]
  Demux1/2 -> Terminator1/1
  Demux1/3 -> Terminator2/1
  Demux2/1 -> [p_rps]
  Demux2/3 -> [r_rps]
  Demux2/2 -> Terminator/1
  [Gamma_deg] -> LongitudinalControl/1(Gamma_deg)
  [AlphaDot_radps] -> LongitudinalControl/2(AlphaDot_rps)
  [r_rps] -> LateroDirectionalControl/3(r_rps)
  [p_rps] -> LateroDirectionalControl/2(p_rps)
  [Phi_deg] -> LateroDirectionalControl/5(Phi_deg)
  [Beta_deg] -> LateroDirectionalControl/4(Beta_deg)
  PhiCmd/1 -> LateroDirectionalControl/1(PhiCmd)
  MachCmd/1 -> EngineControl/1(MachCmd)
  [Mach] -> EngineControl/2(Mach)
  GammaCmd/1 -> LongitudinalControl/4(GammaCmd)
  Q_Dyn_Pa/1 -> [Q_Dyn_Pa]
  [Q_Dyn_Pa] -> LongitudinalControl/3(Q_Dyn_Pa)
  LateroDirectionalControl/2(RudderCmd) -> Trimming2/1(RudderCmd)
  Trimming2/1(DeltaRudderCmd) -> DeltaRudderCmd/1
  LateroDirectionalControl/1(AileronCmd) -> Trimming1/1(AileronCmd)
  Trimming1/1(DeltaAileronCmd) -> DeltaAileronCmd/1
  LongitudinalControl/1(ElevCmd) -> Trimming/1(ElevCmd)
  Trimming/1(DeltaElevCmd) -> DeltaElevCmd/1
  EngineControl/1(EngineCmd) -> Trimming3/1(EngineCmd)
  Trimming3/1(DeltaEngineCmd) -> DeltaEngineCmd/1

== system Logan/ManualControl ==
  Enable : EnablePort
  Constant2 : Constant  Value=0
  Constant3 : Constant  Value=Trimming
  Constant4 : Constant
  Constant5 : Constant
  Dead Zone : DeadZone  LowerValue=-0.05  UpperValue=0.05
  Dead Zone1 : DeadZone  LowerValue=-0.05  UpperValue=0.05
  Gain : Gain  Gain=-45
  Gain1 : Gain  Gain=-5
  Gain3 : Gain  Gain=0.5
  Gain4 : Gain  Gain=-1
  Pilot Joystick : aerolibanimutils/Pilot Joystick  JoystickID=Joystick1  OutputConfiguration=FourAxis  SampleTime=0.01
  Product : Product
  Product1 : Product
  Product3 : Product
  Sum4 : Sum  Inputs=|++
  Switch : Switch  Criteria=u2 > Threshold  Threshold=0.5  SaturateOnIntegerOverflow=off  InputSameDT=off
  Terminator : Terminator
  delta_Stick_Long : Outport
  delta_Stick_Lat : Outport  Port=2
  delta_throttle : Outport  Port=3
  wires:
  Product3/1 -> delta_throttle/1
  Product1/1 -> delta_Stick_Long/1
  Constant4/1 -> Sum4/2
  Gain1/1 -> Product1/2
  Dead Zone1/1 -> Gain1/1
  Gain4/1 -> Sum4/1
  Gain3/1 -> Product3/2
  Constant2/1 -> Switch/1
  Gain/1 -> Product/2
  Pilot Joystick/4 -> Gain4/1  "throttle"
  Dead Zone/1 -> Gain/1
  Pilot Joystick/1 -> Dead Zone/1  "aileron"
  Product/1 -> delta_Stick_Lat/1
  Constant5/1 -> Switch/3
  Pilot Joystick/2 -> Dead Zone1/1  "elevator"
  Sum4/1 -> Gain3/1
  Constant3/1 -> Switch/2
  Switch/1 -> Product1/1, Product3/1, Product/1
  Pilot Joystick/3 -> Terminator/1  "rudder"

== system Logan/Mass Consumption ==
  mass_kg : Inport
  m_dot_fuel : Inport  Port=2
  Constant : Constant  Value=RefMass_kg
  Divide : Product  Inputs=*/
  Fuel_Freeze : Subsystem
  Integrator : Integrator
  Saturation : Saturate  UpperLimit=50000  LowerLimit=18500
  Sum3 : Sum  Inputs=|+-
  Mass_kg : Outport
  MassFraction : Outport  Port=2
  wires:
  Saturation/1 -> Divide/1, Mass_kg/1
  Sum3/1 -> Saturation/1
  mass_kg/1 -> Sum3/1
  m_dot_fuel/1 -> Fuel_Freeze/1(1)
  Divide/1 -> MassFraction/1
  Constant/1 -> Divide/2
  Fuel_Freeze/1(2) -> Integrator/1
  Integrator/1 -> Sum3/2

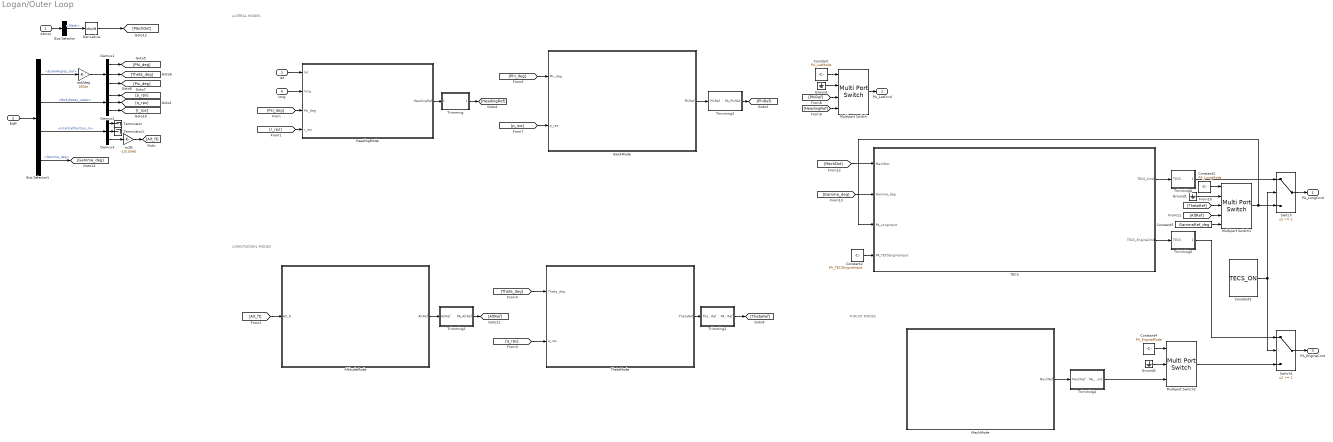
== system Logan/Outer Loop ==
  note: THRUST MODES
  note: LONGITUDINAL MODES
  note: LATERAL MODES
  Atmos : Inport
  EqM : Inport  Port=2
  lat : Inport  Port=3
  long : Inport  Port=4
  AltitudeMode : Subsystem
  BankMode : Subsystem
  Bus Selector : BusSelector  OutputSignals=Mach
  Bus Selector1 : BusSelector  OutputSignals=EulerAngles_rad,BodyRates_radps,IntertialPosition_m,Gamma_deg
  Constant : Constant  Value=PA_LatMode
  Constant1 : Constant  Value=PA_LongMode
  Constant2 : Constant  Value=PA_TECSEngineInput
  Constant3 : Constant  Value=TECS_ON
  Constant4 : Constant  Value=PA_EngineMode
  Constant5 : Constant  Value=GammaRef_deg
  Demux1 : Demux  Outputs=3
  Demux2 : Demux  Outputs=3
  Demux3 : Demux  Outputs=3
  Derivative : Derivative
  Ground : Ground
  Ground1 : Ground
  Ground2 : Ground
  HeadingMode : Subsystem
  MachMode : Subsystem
  Multiport Switch : MultiPortSwitch  DataPortOrder=Zero-based contiguous  DiagnosticForDefault=None  zeroidx=on  SaturateOnIntegerOverflow=off  InputSameDT=off
  Multiport Switch1 : MultiPortSwitch  DataPortOrder=Zero-based contiguous  Inputs=4  DiagnosticForDefault=None  zeroidx=on  SaturateOnIntegerOverflow=off  InputSameDT=off
  Multiport Switch2 : MultiPortSwitch  DataPortOrder=Zero-based contiguous  Inputs=2  DiagnosticForDefault=None  zeroidx=on  SaturateOnIntegerOverflow=off  InputSameDT=off
  Switch : Switch  Threshold=1  SaturateOnIntegerOverflow=off  InputSameDT=off
  Switch1 : Switch  Threshold=1  SaturateOnIntegerOverflow=off  InputSameDT=off
  TECS : Subsystem
  Terminator : Terminator
  Terminator1 : Terminator
  ThetaMode : Subsystem
  Trimming : Subsystem
  Trimming1 : Subsystem
  Trimming2 : Subsystem
  Trimming3 : Subsystem
  Trimming4 : Subsystem
  Trimming5 : Subsystem
  Trimming6 : Subsystem
  m2ft : Gain  Gain=-1/0.3048
  rad2deg : Gain  Gain=180/pi
  PA_LongCmd : Outport
  PA_LatCmd : Outport  Port=2
  PA_EngineCmd : Outport  Port=3
  wires:
  Demux1/2 -> [Theta_deg]
  Demux2/1 -> [p_rps]
  Bus Selector1/2 -> Demux2/1  "<BodyRates_radps>"
  rad2deg/1 -> Demux1/1
  Demux2/2 -> [q_rps]
  Bus Selector1/1 -> rad2deg/1  "<EulerAngles_rad>"
  Demux2/3 -> [r_rps]
  Demux1/1 -> [Phi_deg]
  Demux1/3 -> [Psi_deg]
  EqM/1 -> Bus Selector1/1
  lat/1 -> HeadingMode/1(lat)
  long/1 -> HeadingMode/2(long)
  [Psi_deg] -> HeadingMode/3(Psi_deg)
  [r_rps] -> HeadingMode/4(r_rps)
  Bus Selector1/3 -> Demux3/1  "<IntertialPosition_m>"
  Demux3/3 -> m2ft/1
  Demux3/1 -> Terminator/1
  Demux3/2 -> Terminator1/1
  m2ft/1 -> [Alt_ft]
  [Alt_ft] -> AltitudeMode/1(Alt_ft)
  HeadingMode/1(HeadingRef) -> Trimming/1(HeadingRef)
  [q_rps] -> ThetaMode/2(q_rps)
  [Theta_deg] -> ThetaMode/1(Theta_deg)
  Atmos/1 -> Bus Selector/1
  Bus Selector/1 -> Derivative/1  "<Mach>"
  [Phi_deg] -> BankMode/1(Phi_deg)
  [p_rps] -> BankMode/2(p_rps)
  BankMode/1(PhiRef) -> Trimming3/1(PhiRef)
  ThetaMode/1(ThetaRef) -> Trimming1/1(ThetaRef)
  AltitudeMode/1(AltRef) -> Trimming2/1(AltRef)
  Constant/1 -> Multiport Switch/1
  Multiport Switch/1 -> PA_LatCmd/1
  Ground/1 -> Multiport Switch/2
  Ground1/1 -> Multiport Switch1/2
  Constant1/1 -> Multiport Switch1/1
  Trimming3/1(PA_PhiRef) -> [PhiRef]
  [PhiRef] -> Multiport Switch/3
  Trimming/1(PA_HeadingRef) -> [HeadingRef]
  [HeadingRef] -> Multiport Switch/4
  Trimming1/1(PA_ThetaRef) -> [ThetaRef]
  [ThetaRef] -> Multiport Switch1/3
  Trimming2/1(PA_AltRef) -> [AltRef]
  [AltRef] -> Multiport Switch1/4
  Switch/1 -> PA_LongCmd/1
  TECS/1(TECS_Cmd) -> Trimming6/1(TECS)
  Multiport Switch1/1 -> Switch/3, TECS/3(PA_LongInput)
  Switch1/1 -> PA_EngineCmd/1
  TECS/2(TECS_EngineCmd) -> Trimming5/1(TECS)
  Derivative/1 -> [MachDot]
  [MachDot] -> TECS/1(MachDot)
  Bus Selector1/4 -> [Gamma_deg]  "<Gamma_deg>"
  [Gamma_deg] -> TECS/2(Gamma_deg)
  Constant3/1 -> Switch1/2, Switch/2
  Constant2/1 -> TECS/4(PA_TECSEngineInput)
  Trimming5/1(TECS_EngineCmd) -> Switch1/1
  Trimming6/1(TECS_Cmd) -> Switch/1
  MachMode/1(MachRef) -> Trimming4/1(MachRef)
  Constant4/1 -> Multiport Switch2/1
  Ground2/1 -> Multiport Switch2/2
  Multiport Switch2/1 -> Switch1/3
  Trimming4/1(PA_EngineCmd) -> Multiport Switch2/3
  Constant5/1 -> Multiport Switch1/5

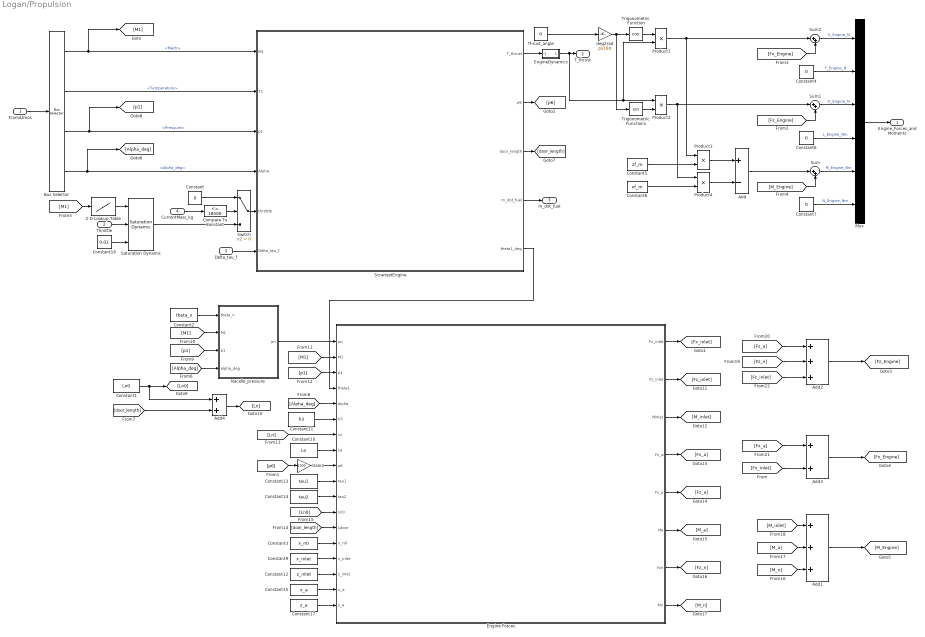
== system Logan/Propulsion ==
  FromAtmos : Inport
  Throttle : Inport  Port=2
  Delta_tau_f : Inport  Port=3
  CurrentMass_kg : Inport  Port=4
  2-D Lookup Table : Lookup_n-D  NumberOfTableDimensions=1  BreakpointsForDimension1=[4;5;6;7;10]  BreakpointsForDimension2=[1:3]  Table=[0.3;0.4;0.5;0.7;1]  InternalRulePriority=Speed  RndMeth=Simplest
  Add : Sum  Inputs=+-
  Add1 : Sum  Inputs=+++
  Add2 : Sum  Inputs=+++
  Add3 : Sum
  Add4 : Sum
  Bus Selector : BusSelector  OutputSignals=Mach,Temperature,Pressure,Alpha_deg
  Compare To Constant : simulink/Logic and Bit Operations/Compare To Constant  relop=<=  const=18500  OutDataTypeStr=boolean
  Constant{,4,6..7} (4 alike) : Constant  Value=0
  Constant1 : Constant  Value=Ln0
  Constant10 : Constant  Value=La
  Constant11 : Constant  Value=h3
  Constant12 : Constant  Value=z_inlet
  Constant13 : Constant  Value=tau1
  Constant14 : Constant  Value=tau2
  Constant15 : Constant  Value=x_a
  Constant16 : Constant  Value=0.01
  Constant17 : Constant  Value=z_a
  Constant2 : Constant  Value=theta_n
  Constant3 : Constant  Value=x_n0
  Constant5 : Constant  Value=zf_m
  Constant8 : Constant  Value=xf_m
  Constant9 : Constant  Value=x_inlet
  Engine Forces : MATLAB Function  TreatAsAtomicUnit=on
  EngineDynamics : Subsystem
  Gain3 : Gain  Gain=1000
  Mux : Mux  Inputs=6
  Nacelle_pressure : MATLAB Function  TreatAsAtomicUnit=on
  Product{1..4} (4 alike) : Product
  Saturation Dynamic : simulink/Discontinuities/Saturation Dynamic  OutMin=[]  OutMax=[]  OutDataTypeStr=Inherit: Same as second input  OutDataType=fixdt(1, 16)  OutScaling=2^-10  DoSatur=off
  ScramjetEngine : Subsystem
  Sum : Sum  Inputs=|++
  Sum1 : Sum  Inputs=|++
  Sum2 : Sum  Inputs=|++
  Switch : Switch  Criteria=u2 > Threshold  SaturateOnIntegerOverflow=off  InputSameDT=off
  Thrust_angle : Constant  Value=0
  Trigonometric Function : Trigonometry  Operator=cos
  Trigonometric Function1 : Trigonometry
  deg2rad : Gain  Gain=pi/180
  Engine_Forces_and Moments : Outport
  T_thrust : Outport  Port=2
  m_dot_fuel : Outport  Port=3
  wires:
  Constant8/1 -> Product4/2
  Constant4/1 -> Mux/2  "Y_Engine_N"
  Product1/1 -> Product3/1, Sum2/1
  deg2rad/1 -> Trigonometric Function1/1, Trigonometric Function/1
  Product2/1 -> Sum1/1, Product4/1
  FromAtmos/1 -> Bus Selector/1
  Constant7/1 -> Mux/6  "N_Engine_Nm"
  Constant6/1 -> Mux/4  "L_Engine_Nm"
  Product4/1 -> Add/2
  Constant5/1 -> Product3/2
  Product3/1 -> Add/1
  Trigonometric Function1/1 -> Product2/2
  Bus Selector/1 -> ScramjetEngine/1(M1), [M1]  "<Mach>"
  Mux/1 -> Engine_Forces_and Moments/1
  Bus Selector/3 -> [p1], ScramjetEngine/3(p1)  "<Pressure>"
  Bus Selector/2 -> ScramjetEngine/2(T1)  "<Temperature>"
  Thrust_angle/1 -> deg2rad/1
  EngineDynamics/1(T_thrust) -> Product1/2, Product2/1, T_thrust/1
  Delta_tau_f/1 -> ScramjetEngine/6(Delta_tau_f)
  Bus Selector/4 -> [Alpha_deg], ScramjetEngine/4(Alpha)  "<Alpha_deg>"
  ScramjetEngine/1(T_thrust) -> EngineDynamics/1(Thrust)
  Constant3/1 -> Engine Forces/14(x_n0)
  Constant11/1 -> Engine Forces/6(h3)
  ScramjetEngine/2(p6) -> [p6]
  [p6] -> Gain3/1
  Constant10/1 -> Engine Forces/8(La)
  ScramjetEngine/5(theta1_deg) -> Engine Forces/4(theta1)
  Constant14/1 -> Engine Forces/11(tau2)
  Gain3/1 -> Engine Forces/9(p6)
  Add/1 -> Sum/1
  Sum/1 -> Mux/5  "M_Engine_Nm"
  Sum2/1 -> Mux/1  "X_Engine_N"
  Sum1/1 -> Mux/3  "Z_Engine_N"
  2-D Lookup Table/1 -> Saturation Dynamic/1
  Constant16/1 -> Saturation Dynamic/3
  [M1] -> 2-D Lookup Table/1
  [Alpha_deg] -> Nacelle_pressure/4(alpha_deg)
  ScramjetEngine/3(door_length) -> [door_length]
  Trigonometric Function/1 -> Product1/1
  [Alpha_deg] -> Engine Forces/5(alpha)
  [p1] -> Nacelle_pressure/3(p1)
  [M1] -> Nacelle_pressure/2(M1)
  Nacelle_pressure/1(pn) -> Engine Forces/1(pn)
  [M1] -> Engine Forces/2(M1)
  [p1] -> Engine Forces/3(p1)
  [Ln] -> Engine Forces/7(Ln)
  Constant1/1 -> Add4/1, [Ln0]
  [door_length] -> Engine Forces/13(Ldoor)
  [Ln0] -> Engine Forces/12(Ln0)
  Add4/1 -> [Ln]
  [door_length] -> Add4/2
  Constant9/1 -> Engine Forces/15(x_inlet)
  Constant12/1 -> Engine Forces/16(z_inlet)
  Constant13/1 -> Engine Forces/10(tau1)
  Constant15/1 -> Engine Forces/17(x_a)
  Constant17/1 -> Engine Forces/18(z_a)
  Engine Forces/1(Fx_inlet) -> [Fx_inlet]
  Engine Forces/2(Fz_inlet) -> [Fz_inlet]
  Engine Forces/3(Minlet) -> [M_inlet]
  Engine Forces/4(Fx_a) -> [Fx_a]
  Engine Forces/5(Fz_a) -> [Fz_a]
  Engine Forces/6(Ma) -> [M_a]
  Engine Forces/7(Fzn) -> [Fz_n]
  Engine Forces/8(Mn) -> [M_n]
  [M_n] -> Add1/3
  [M_a] -> Add1/2
  [M_inlet] -> Add1/1
  [Fx_a] -> Add3/1
  [Fz_a] -> Add2/1
  [Fz_n] -> Add2/2
  [Fz_inlet] -> Add2/3
  [Fx_inlet] -> Add3/2
  Add2/1 -> [Fz_Engine]
  Add3/1 -> [Fx_Engine]
  Add1/1 -> [M_Engine]
  ScramjetEngine/4(m_dot_fuel) -> m_dot_fuel/1
  CurrentMass_kg/1 -> Compare To Constant/1
  Compare To Constant/1 -> Switch/2
  Constant/1 -> Switch/1
  Saturation Dynamic/1 -> Switch/3
  Throttle/1 -> Saturation Dynamic/2
  Constant2/1 -> Nacelle_pressure/1(theta_n)
  [Fz_Engine] -> Sum1/2
  [M_Engine] -> Sum/2
  [Fx_Engine] -> Sum2/2
  Switch/1 -> ScramjetEngine/5(throttle)

== system Logan/SurfaceActuators ==
  ElevatorCmd : Inport
  AileronCmd : Inport  Port=2
  RudderCmd : Inport  Port=3
  Add : Sum  Inputs=-+
  Add1 : Sum
  L_ElevActuator : aerolibactuator/Nonlinear Second-Order Actuator  wn_fin=20  z_fin=5  fin_max=250  fin_min=-250  fin_maxrate=120  fin_act_0=Aileron_init  fin_act_vel=0
  R_ElevActuator : aerolibactuator/Nonlinear Second-Order Actuator  wn_fin=20  z_fin=5  fin_max=250  fin_min=-250  fin_maxrate=120  fin_act_0=Elevator_init  fin_act_vel=0
  RudderActuator : aerolibactuator/Nonlinear Second-Order Actuator  wn_fin=20  z_fin=5  fin_max=250  fin_min=-250  fin_maxrate=120  fin_act_0=Rudder_init  fin_act_vel=0
  Saturation3 : Saturate  UpperLimit=15  LowerLimit=-15
  Saturation4 : Saturate  UpperLimit=40  LowerLimit=-40
  Saturation5 : Saturate  UpperLimit=40  LowerLimit=-40
  To Workspace3 : ToWorkspace  VariableName=L_ElevActuator_Actual  SampleTime=-1
      settings: Save2DSignal=2-D array (concatenate along first dimension)
  To Workspace4 : ToWorkspace  VariableName=RudderActuator_Actual  SampleTime=-1
      settings: Save2DSignal=2-D array (concatenate along first dimension)
  To Workspace5 : ToWorkspace  VariableName=R_ElevActuator_Actual  SampleTime=-1
      settings: Save2DSignal=2-D array (concatenate along first dimension)
  R_Elevon_deg : Outport
  L_Elevon_deg : Outport  Port=2
  RudderCmd_deg : Outport  Port=3
  wires:
  Add1/1 -> Saturation4/1
  RudderActuator/1 -> To Workspace4/1, RudderCmd_deg/1
  Saturation4/1 -> R_ElevActuator/1
  Saturation3/1 -> RudderActuator/1
  ElevatorCmd/1 -> Add1/1, Add/2
  R_ElevActuator/1 -> To Workspace5/1, R_Elevon_deg/1
  RudderCmd/1 -> Saturation3/1
  Add/1 -> Saturation5/1
  Saturation5/1 -> L_ElevActuator/1
  L_ElevActuator/1 -> To Workspace3/1, L_Elevon_deg/1
  AileronCmd/1 -> Add/1, Add1/2

== system Logan/Aero/L_50%2CG ==
  Y_Aero_N : Inport
  Z_Aero_N : Inport  Port=2
  Lb_Nm : Inport  Port=3
  Add : Sum  Inputs=--+
  Product7 : Product
  Product8 : Product
  y_CG_m : Constant  Value=y_cg
  z_CG_m : Constant  Value=z_cg
  L_Aero_Nm : Outport
  wires:
  Z_Aero_N/1 -> Product8/1
  Y_Aero_N/1 -> Product7/1
  y_CG_m/1 -> Product8/2
  Add/1 -> L_Aero_Nm/1  "L_Aero_Nm"
  Lb_Nm/1 -> Add/3
  Product7/1 -> Add/1
  Product8/1 -> Add/2
  z_CG_m/1 -> Product7/2

== system Logan/Aero/M_50%2CG ==
  X_Aero_N : Inport
  Z_Aero_N : Inport  Port=2
  CG_mac : Inport  Port=3
  Mb_Nm : Inport  Port=4
  Add : Sum  Inputs=-++
  Fcn : Fcn  Expr=(u(1) -0.5)*c
  Product5 : Product
  Product6 : Product
  z_CG_m : Constant  Value=z_cg
  M_Aero_Nm : Outport
  wires:
  z_CG_m/1 -> Product6/2
  Product6/1 -> Add/2
  Add/1 -> M_Aero_Nm/1  "M_Aero_Nm"
  X_Aero_N/1 -> Product6/1
  Z_Aero_N/1 -> Product5/1
  Product5/1 -> Add/1
  Fcn/1 -> Product5/2
  CG_mac/1 -> Fcn/1
  Mb_Nm/1 -> Add/3

== system Logan/Aero/N_50%2CG ==
  X_Aero_N : Inport
  Y_Aero_N : Inport  Port=2
  CG_mac : Inport  Port=3
  Nb_Nm : Inport  Port=4
  Add : Sum  Inputs=+++
  Fcn : Fcn  Expr=(u(1) -0.5)*c
  Product6 : Product
  Product7 : Product
  y_CG_m : Constant  Value=y_cg
  N_Aero_Nm : Outport
  wires:
  Product7/1 -> Add/2
  y_CG_m/1 -> Product7/2
  Add/1 -> N_Aero_Nm/1  "N_Aero_Nm"
  Nb_Nm/1 -> Add/3
  Fcn/1 -> Product6/2
  Product6/1 -> Add/1
  X_Aero_N/1 -> Product7/1
  CG_mac/1 -> Fcn/1
  Y_Aero_N/1 -> Product6/1

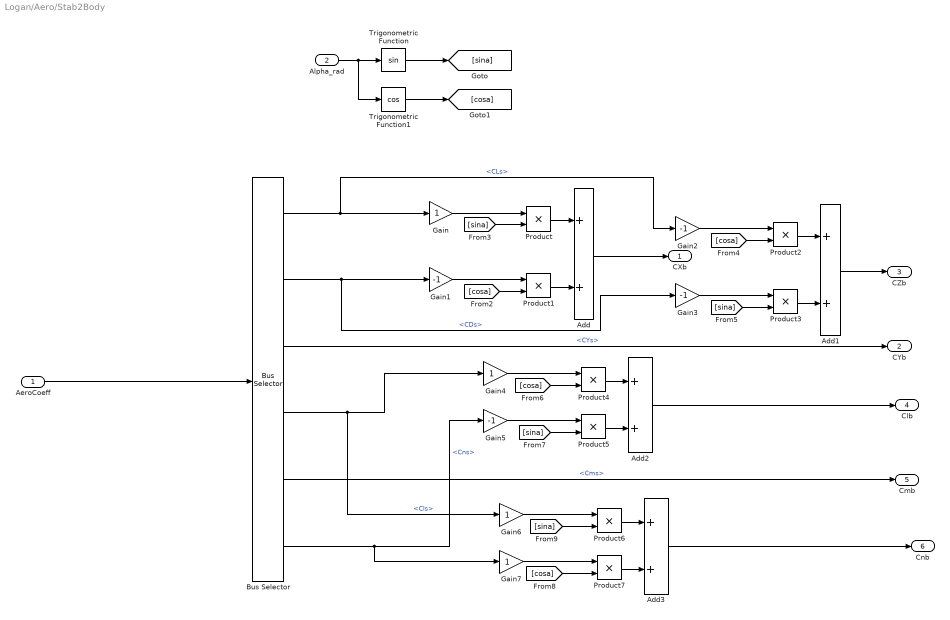
== system Logan/Aero/Stab2Body ==
  AeroCoeff : Inport
  Alpha_rad : Inport  Port=2
  Add{,1..3} (4 alike) : Sum
  Bus Selector : BusSelector  OutputSignals=CLs,CDs,CYs,Cls,Cms,Cns
  Gain{,4,6..7} (4 alike) : Gain
  Gain{1..3,5} (4 alike) : Gain  Gain=-1
  Product{,1..7} (8 alike) : Product
  Trigonometric Function : Trigonometry
  Trigonometric Function1 : Trigonometry  Operator=cos
  CXb : Outport
  CYb : Outport  Port=2
  CZb : Outport  Port=3
  Clb : Outport  Port=4
  Cmb : Outport  Port=5
  Cnb : Outport  Port=6
  wires:
  AeroCoeff/1 -> Bus Selector/1
  Alpha_rad/1 -> Trigonometric Function1/1, Trigonometric Function/1
  Trigonometric Function/1 -> [sina]
  Trigonometric Function1/1 -> [cosa]
  [sina] -> Product/2
  Bus Selector/1 -> Gain2/1, Gain/1  "<CLs>"
  Gain/1 -> Product/1
  [cosa] -> Product1/2
  Bus Selector/2 -> Gain3/1, Gain1/1  "<CDs>"
  Gain1/1 -> Product1/1
  Product1/1 -> Add/2
  Product/1 -> Add/1
  Add/1 -> CXb/1
  Gain2/1 -> Product2/1
  Gain3/1 -> Product3/1
  Product3/1 -> Add1/2
  Product2/1 -> Add1/1
  [sina] -> Product3/2
  [cosa] -> Product2/2
  Bus Selector/3 -> CYb/1  "<CYs>"
  Bus Selector/5 -> Cmb/1  "<Cms>"
  [cosa] -> Product4/2
  Gain4/1 -> Product4/1
  Gain5/1 -> Product5/1
  Product4/1 -> Add2/1
  Add2/1 -> Clb/1
  Product5/1 -> Add2/2
  Bus Selector/4 -> Gain6/1, Gain4/1  "<Cls>"
  Bus Selector/6 -> Gain7/1, Gain5/1  "<Cns>"
  [sina] -> Product5/2
  [sina] -> Product6/2
  Gain6/1 -> Product6/1
  Gain7/1 -> Product7/1
  Product6/1 -> Add3/1
  Add3/1 -> Cnb/1
  Product7/1 -> Add3/2
  [cosa] -> Product7/2
  Add1/1 -> CZb/1

== system Logan/Atmospheric/TAS2CAS ==
  Pressure_Pa : Inport
  Mach : Inport  Port=2
  (Gamma-1)/2 : Gain  Gain=(1.4-1)/2
  (Gamma-1)/Gamma : Constant  Value=(1.4-1)/1.4
  2*a0^2/(Gamma-1) : Gain  Gain=(2*340.262^2)/(1.4-1)
  Add2 : Sum
  Add3 : Sum  Inputs=+-
  Add4 : Sum
  Add5 : Sum  Inputs=+-
  Constant2 : Constant
  Divide5 : Product  Inputs=**
  Divide6 : Product  Inputs=*/
  Gamma/(Gamma-1) : Constant  Value=1.4/(1.4-1)
  Math Function2 : Math  Operator=square  SignedPower=on
  Math Function3 : Math  Operator=pow  SignedPower=on
  Math Function4 : Math  Operator=pow  SignedPower=on
  P0_Pa : Constant  Value=101325
  Sqrt2 : Sqrt
  CAS_mps : Outport
  wires:
  Sqrt2/1 -> CAS_mps/1
  2*a0^2/(Gamma-1)/1 -> Sqrt2/1
  Add5/1 -> 2*a0^2/(Gamma-1)/1
  Math Function4/1 -> Add5/1
  (Gamma-1)/Gamma/1 -> Math Function4/2
  Add4/1 -> Math Function4/1
  Divide6/1 -> Add4/1
  P0_Pa/1 -> Divide6/2
  Divide5/1 -> Divide6/1  "pt-ps"
  Pressure_Pa/1 -> Divide5/1
  Math Function3/1 -> Add3/1
  Add3/1 -> Divide5/2
  Gamma/(Gamma-1)/1 -> Math Function3/2
  Add2/1 -> Math Function3/1
  Constant2/1 -> Add5/2, Add4/2, Add3/2, Add2/2
  (Gamma-1)/2/1 -> Add2/1
  Mach/1 -> Math Function2/1
  Math Function2/1 -> (Gamma-1)/2/1

== system Logan/EqM/BodyRates ==
  InertiaTensor_kgm2 : Inport
  Moments_Nm : Inport  Port=2
  CrossProduct : Subsystem
  Demux : Demux  Outputs=3
  Divide : Product  Inputs=/*  Multiplication=Matrix(*)
  Mux : Mux  Inputs=3
  Product : Product  Multiplication=Matrix(*)
  Sum : Sum  Inputs=|-+
  p_radps : Integrator  ContinuousStateAttributes='p_radps'
  q_radps : Integrator  ContinuousStateAttributes='q_radps'
  r_radps : Integrator  ContinuousStateAttributes='r_radps'
  BodyRates_radps : Outport
  wires:
  Divide/1 -> Demux/1
  Demux/2 -> q_radps/1
  Demux/3 -> r_radps/1
  Demux/1 -> p_radps/1
  InertiaTensor_kgm2/1 -> Product/1, Divide/1
  q_radps/1 -> Mux/2  "q_radps"
  CrossProduct/1(C) -> Sum/1
  Moments_Nm/1 -> Sum/2
  Product/1 -> CrossProduct/2(B)
  p_radps/1 -> Mux/1  "p_radps"
  Sum/1 -> Divide/2
  Mux/1 -> Product/2, CrossProduct/1(A), BodyRates_radps/1
  r_radps/1 -> Mux/3  "r_radps"

== system Logan/EqM/BodyVelocities ==
  Forces_N : Inport
  Mass_kg : Inport  Port=2
  BodyRates_radps : Inport  Port=3
  Add : Sum  Inputs=+-
  CrossProduct : Subsystem
  Demux : Demux  Outputs=3
  Divide : Product  Inputs=*/
  Mux : Mux  Inputs=3
  u_mps : Integrator  ContinuousStateAttributes='u_mps'
  v_mps : Integrator  ContinuousStateAttributes='v_mps'
  w_mps : Integrator  ContinuousStateAttributes='w_mps'
  VB_mps : Outport
  wires:
  Mass_kg/1 -> Divide/2
  u_mps/1 -> Mux/1
  Demux/3 -> w_mps/1
  Demux/2 -> v_mps/1
  w_mps/1 -> Mux/3
  v_mps/1 -> Mux/2
  Demux/1 -> u_mps/1
  CrossProduct/1(C) -> Add/2
  BodyRates_radps/1 -> CrossProduct/1(A)
  Mux/1 -> VB_mps/1, CrossProduct/2(B)
  Forces_N/1 -> Divide/1
  Add/1 -> Demux/1  "VB_dot_mps2"
  Divide/1 -> Add/1

== system Logan/EqM/EulerAngles ==
  BodyRates_radps : Inport
  Demux : Demux  Outputs=3
  EulerRates : Subsystem
  LBE_rotation : Subsystem
  Mux1 : Mux  Inputs=3
  PHI_rad : Integrator  ContinuousStateAttributes='PHI_rad'
  PSI_rad : Integrator  ContinuousStateAttributes='PSI_rad'
  THETA_rad : Integrator  ContinuousStateAttributes='THETA_rad'
  LBE : Outport
  EulerAngles_rad : Outport  Port=2
  wires:
  BodyRates_radps/1 -> EulerRates/1(BodyRates_radps)
  LBE_rotation/1(LBE) -> LBE/1
  EulerRates/1(EulerRates_radsps2) -> Demux/1
  Demux/1 -> PHI_rad/1
  Mux1/1 -> LBE_rotation/1(EulerAngles_rad), EulerAngles_rad/1, EulerRates/2(EulerAngles_rad)
  PSI_rad/1 -> Mux1/3
  THETA_rad/1 -> Mux1/2
  PHI_rad/1 -> Mux1/1
  Demux/3 -> PSI_rad/1
  Demux/2 -> THETA_rad/1
